simulink model "sd2"  (Simulink 2.20)
settings: Solver=FixedStepDiscrete  StartTime=0.0  StopTime=6e-3  FixedStep=Ts  MaxStep=3.90625e-06  RelTol=1e-3  AbsTol=1e-3
values from neighbouring files (symbols this model uses):
  alfa = (1e3-1)/1e3    (= 0.999)    [SD2script.m]    (also in SD2script_falsi.m)
  Amax = 1.35    [SD2script.m]    (also in SD2script_falsi.m)
  Ampl = 0.5-pi/256    (= 0.487728153697)    [SD2script.m]    (also in SD2script_falsi.m)
  b = 0.5    [SD2script.m]    (also in SD2script_falsi.m)
  b2 = 0.5    [SD2script.m]    (also in SD2script_falsi.m)
  Cf = 5e-12    [SD2script.m]    (also in SD2script_falsi.m)
  delta = 4e-9    (= 4e-09)    [SD2script.m]    (also in SD2script_falsi.m)
  finrad = Fin*2*pi    (= 12988.5221272)    [SD2script.m]    (also in SD2script_falsi.m)
  GBW = 150e6    (= 150000000)    [SD2script.m]    (also in SD2script_falsi.m)
  k = 1.38e-23    [SD2script.m]    (also in SD2script_falsi.m)
  noise1 = 10e-6    (= 1e-05)    [SD2script.m]    (also in SD2script_falsi.m)
  sr = 20e6    (= 20000000)    [SD2script.m]    (also in SD2script_falsi.m)
  Temp = 300    [SD2script.m]    (also in SD2script_falsi.m)
  Ts = 1/Fs    (= 8.85770975057e-08)    [SD2script.m]    (also in SD2script_falsi.m)
  Vref = 1    [SD2script.m]    (also in SD2script_falsi.m)
undefined symbols (not defined in the file or in its folder): clock, slew
CloseFcn:
  | ;slview('closediagram',bdroot);
settings Model: SaveTime=off  SaveOutput=off  ConsistencyChecking=off  RTWPlaceOutputsASAP=off  RTWTemplateMakefile=grt.tmf

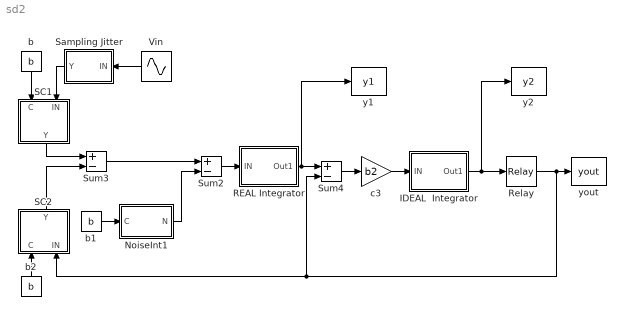
== system sd2 ==
  IDEAL  Integrator : Subsystem  mask(Integrator){Amax=Amax, Ts=Ts}
      mask prompts: Amax "Saturation"; Ts "Sample Time:"
      mask help:
      | Real discrete integrator with delay.
      | Models op-amp saturation and slew rate.
      mask Help:
      | Parameters:
      | Ts:       Sample time
      | G:         Finite op-amp gain (ideal op-amp G=1)
      | Amax:  Saturation value
      | sr:       slew rate in V/s
      mask Display: dpoly([0 1], [1 -1], 'z-')
  NoiseInt1 : Subsystem  mask(OpAmp Noise){seed=sum(clock)^1/111, Ts=Ts, noise=noise1}
      mask prompts: seed "Random Number Seed:"; Ts "Sample Time:"; noise "Op-amp Noise Std. Dev.:"
      mask Display: disp('OpNoise')
  REAL Integrator : Subsystem  mask(Integrator){Ts=Ts, alfa=alfa, Amax=Amax, sr=sr, GBW=GBW}
      mask prompts: Ts "Sample Time:"; alfa "Finite Gain:"; Amax "Saturation:"; sr "Slew Rate:"; GBW "Gain-Bandwidth"
      mask help:
      | Real discrete integrator with delay.
      | Models op-amp saturation and slew rate.
      mask Help:
      | Parameters:
      | Ts:       Sample time
      | G:         Finite op-amp gain (ideal op-amp G=1)
      | Amax:  Saturation value
      | sr:       slew rate in V/s
      mask Display: dpoly([0 1], [1 -1], 'z-')
  Relay : Relay  OnSwitchValue=eps  OffSwitchValue=-eps  OnOutputValue=Vref  OffOutputValue=-Vref
  SC1 : Subsystem  Orientation=down  mask(kT/C Noise){Ts=Ts, Ci=Cf, Temp=Temp, k=k, seed=sum(clock)}
      mask prompts: Ts "Sample Time:"; Ci "Integrating Capacitance:"; Temp "Absolute Temperature:"; k "Boltzman Constant:"; seed "Random Number Seed:"
      mask help:
      | Models the kT/Cs noise of a switched capacitance Cs.
      | IN input: the input signal line
      | C input:   accepts the coefficient WITH SIGN (Cs/Ci)
      mask Help:
      | Block parameters:
      | Ts:        Sample time
      | Ci:        Integrating Capacitance
      | Temp:   Absolute Temperature in Kelvin
      | k:         Boltzmann Constant
      | seed:    Initial seed for random number generator
      | Outputs the noisy signal.
      mask Display: disp('kT/C')
  SC2 : Subsystem  Orientation=up  mask(kT/C Noise){Ts=Ts, Ci=Cf, Temp=Temp, k=k, seed=2.11*sum(clock)}
      mask prompts: Ts "Sample Time:"; Ci "Integrating Capacitance:"; Temp "Absolute Temperature:"; k "Boltzman Constant:"; seed "Random Number Seed:"
      mask help:
      | Models the kT/Cs noise of a switched capacitance Cs.
      | IN input: the input signal line
      | C input:   accepts the coefficient WITH SIGN (Cs/Ci)
      mask Help:
      | Block parameters:
      | Ts:        Sample time
      | Ci:        Integrating Capacitance
      | Temp:   Absolute Temperature in Kelvin
      | k:         Boltzmann Constant
      | seed:    Initial seed for random number generator
      | Outputs the noisy signal.
      mask Display: disp('kT/C')
  Sampling Jitter : Subsystem  Orientation=left  mask(Jitter){Ts=Ts, delta=delta, seed=(sum(clock))^3.33}
      mask prompts: Ts "Sample Time:"; delta "Sampling Jitter:"; seed "Random Number Seed:"
      mask help:
      | Models the kT/Cs noise of a switched capacitance Cs.
      | IN input: the input signal line
      | C input:   accepts the coefficient WITH SIGN (Cs/Ci)
      mask Help:
      | Block parameters:
      | Ts:        Sample time
      | Ci:        Integrating Capacitance
      | Temp:   Absolute Temperature in Kelvin
      | k:         Boltzmann Constant
      | seed:    Initial seed for random number generator
      | Outputs the noisy signal.
      mask Display: disp('Jitter')
  Sum2 : Sum  Inputs=+-
  Sum3 : Sum  Inputs=+-
  Sum4 : Sum  Inputs=+-
  Vin : Sin  Orientation=left  Amplitude=Ampl  Frequency=finrad  Phase=0  SampleTime=0
  b : Constant  Orientation=down  Value=b
  b1 : Constant  Value=b
  b2 : Constant  Orientation=up  Value=b
  c3 : Gain  Gain=b2
  y1 : ToWorkspace  VariableName=y1  SampleTime=-1
  y2 : ToWorkspace  VariableName=y2  SampleTime=-1
  yout : ToWorkspace  VariableName=yout  SampleTime=-1
  wires:
  Sum2/1 -> REAL Integrator/1(IN)
  Sum4/1 -> c3/1
  c3/1 -> IDEAL  Integrator/1(IN)
  NoiseInt1/1(N) -> Sum2/2
  b1/1 -> NoiseInt1/1(C)
  Sum3/1 -> Sum2/1
  SC1/1(Y) -> Sum3/1
  b/1 -> SC1/1(C)
  SC2/1(Y) -> Sum3/2
  Sampling Jitter/1(Y) -> SC1/2(IN)
  b2/1 -> SC2/1(C)
  REAL Integrator/1(Out1) -> Sum4/1, y1/1
  Relay/1 -> yout/1, Sum4/2, SC2/2(IN)
  IDEAL  Integrator/1(Out1) -> y2/1, Relay/1
  Vin/1 -> Sampling Jitter/1(IN)

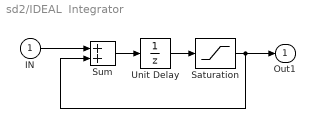
== system sd2/IDEAL  Integrator ==
  IN : Inport  Port=1  PortWidth=-1  SampleTime=-1
  Saturation : Saturate  UpperLimit=Amax  LowerLimit=-Amax
  Sum : Sum  Inputs=++
  Unit Delay : UnitDelay  X0=0  SampleTime=Ts
  Out1 : Outport  Port=1
  wires:
  Sum/1 -> Unit Delay/1
  IN/1 -> Sum/1
  Unit Delay/1 -> Saturation/1
  Saturation/1 -> Out1/1, Sum/2

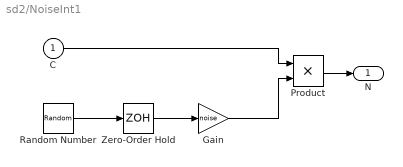
== system sd2/NoiseInt1 ==
  C : Inport  Port=1  PortWidth=-1  SampleTime=-1
  Gain : Gain  Gain=noise
  Product : Product  Inputs=2
  Random Number : RandomNumber  Mean=0  Variance=1  Seed=seed  SampleTime=Ts
  Zero-Order Hold : ZeroOrderHold  SampleTime=Ts
  N : Outport  Port=1  InitialOutput=0
  wires:
  Random Number/1 -> Zero-Order Hold/1
  Zero-Order Hold/1 -> Gain/1
  Product/1 -> N/1
  Gain/1 -> Product/2
  C/1 -> Product/1

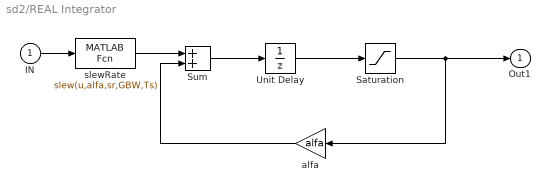
== system sd2/REAL Integrator ==
  IN : Inport  Port=1  PortWidth=-1  SampleTime=-1
  Saturation : Saturate  UpperLimit=Amax  LowerLimit=-Amax
  Sum : Sum  Inputs=++
  Unit Delay : UnitDelay  X0=0  SampleTime=Ts
  alfa : Gain  Orientation=left  Gain=alfa
  slewRate : MATLABFcn  MATLABFcn=slew(u,alfa,sr,GBW,Ts)  OutputWidth=-1
  Out1 : Outport  Port=1
  wires:
  Sum/1 -> Unit Delay/1
  Unit Delay/1 -> Saturation/1
  Saturation/1 -> Out1/1, alfa/1
  IN/1 -> slewRate/1
  slewRate/1 -> Sum/1
  alfa/1 -> Sum/2

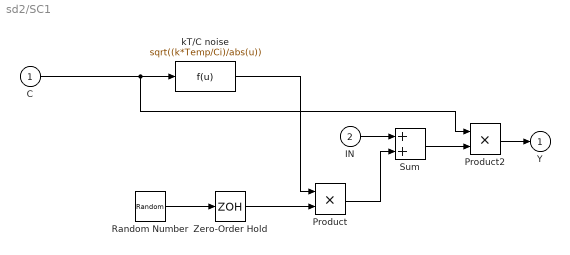
== system sd2/SC1 ==
  C : Inport  Port=1  PortWidth=-1  SampleTime=-1
  IN : Inport  Port=2  PortWidth=-1  SampleTime=-1
  Product : Product  Inputs=2
  Product2 : Product  Inputs=2
  Random Number : RandomNumber  Mean=0  Variance=1  Seed=seed  SampleTime=Ts
  Sum : Sum  Inputs=++
  Zero-Order Hold : ZeroOrderHold  SampleTime=Ts
  kT/C noise : Fcn  Expr=sqrt((k*Temp/Ci)/abs(u))
  Y : Outport  Port=1  InitialOutput=0
  wires:
  Random Number/1 -> Zero-Order Hold/1
  C/1 -> Product2/1, kT/C noise/1
  Zero-Order Hold/1 -> Product/2
  kT/C noise/1 -> Product/1
  Sum/1 -> Product2/2
  IN/1 -> Sum/1
  Product2/1 -> Y/1
  Product/1 -> Sum/2

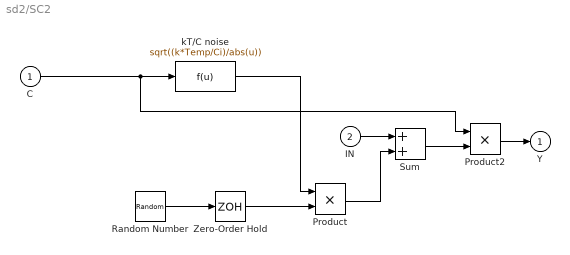
== system sd2/SC2 ==
  C : Inport  Port=1  PortWidth=-1  SampleTime=-1
  IN : Inport  Port=2  PortWidth=-1  SampleTime=-1
  Product : Product  Inputs=2
  Product2 : Product  Inputs=2
  Random Number : RandomNumber  Mean=0  Variance=1  Seed=seed  SampleTime=Ts
  Sum : Sum  Inputs=++
  Zero-Order Hold : ZeroOrderHold  SampleTime=Ts
  kT/C noise : Fcn  Expr=sqrt((k*Temp/Ci)/abs(u))
  Y : Outport  Port=1  InitialOutput=0
  wires:
  Random Number/1 -> Zero-Order Hold/1
  C/1 -> Product2/1, kT/C noise/1
  Zero-Order Hold/1 -> Product/2
  kT/C noise/1 -> Product/1
  Sum/1 -> Product2/2
  IN/1 -> Sum/1
  Product2/1 -> Y/1
  Product/1 -> Sum/2

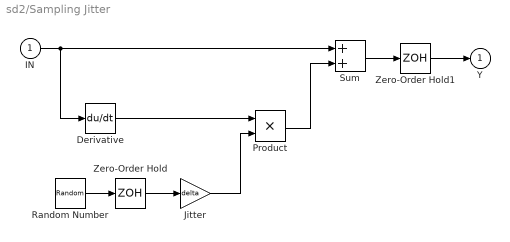
== system sd2/Sampling Jitter ==
  IN : Inport  Port=1  PortWidth=-1  SampleTime=-1
  Derivative : Derivative
  Jitter : Gain  Gain=delta
  Product : Product  Inputs=2
  Random Number : RandomNumber  Mean=0  Variance=1  Seed=seed  SampleTime=Ts
  Sum : Sum  Inputs=++
  Zero-Order Hold : ZeroOrderHold  SampleTime=Ts
  Zero-Order Hold1 : ZeroOrderHold  SampleTime=Ts
  Y : Outport  Port=1  InitialOutput=0
  wires:
  IN/1 -> Sum/1, Derivative/1
  Random Number/1 -> Zero-Order Hold/1
  Derivative/1 -> Product/1
  Zero-Order Hold/1 -> Jitter/1
  Jitter/1 -> Product/2
  Product/1 -> Sum/2
  Sum/1 -> Zero-Order Hold1/1
  Zero-Order Hold1/1 -> Y/1
